simulink model "ESS_3P_2L_220kW_for_LS_Project"  (R2023b)
settings: Solver=VariableStepAuto  StartTime=0.0  StopTime=3  RelTol=1e-3
InitFcn:
  | %Initialization_for_ESS_3P_2L_220kW;
  | Initialization_for_ESS_3P_2L_220kW;
values from neighbouring files (symbols this model uses):
  C_grid = 54e-6    (= 5.4e-05)    [Initialization_for_ESS_3P_2L_220kW.m]    (also in Initialization_for_Testbench.m = 4.5e-05)
  Cdc = 180e-6    (= 0.00018)    [CurrentLoop.m]    (also in Initialization_for_ESS_3P_2L_220kW.m; Initialization_for_Testbench.m)
  Fnom_Grid = 50    [CurrentLoop.m]    (also in Initialization_for_ESS_3P_2L_220kW.m; Initialization_for_Testbench.m)
  Gain_for_ActiveDamping = 1    [Initialization_for_Testbench.m]
  Inom = Pnom/sqrt(3)/Unom_Grid    [CurrentLoop.m]    (also in Initialization_for_ESS_3P_2L_220kW.m; Initialization_for_Testbench.m)
  Ki_Edq = Kp_Edq*2*pi*10    (= 18.8495559215)    [Initialization_for_ESS_3P_2L_220kW.m]
  Ki_Idq = Kp_Idq*2*pi*10    (= 157.913670417)    [Initialization_for_ESS_3P_2L_220kW.m]    (also in Initialization_for_Testbench.m = 1.26330936334)
  Kp_Edq = 0.3    [Initialization_for_ESS_3P_2L_220kW.m]
  Kp_Idq = L_grid*2*pi*2000    (= 2.51327412287)    [Initialization_for_ESS_3P_2L_220kW.m]    (also in Initialization_for_Testbench.m = 2.0106192983)
  L_grid = 200e-6    (= 0.0002)    [Initialization_for_ESS_3P_2L_220kW.m]    (also in Initialization_for_Testbench.m)
  Pnom = 220e3    (= 220000)    [CurrentLoop.m]    (also in Initialization_for_ESS_3P_2L_220kW.m; Initialization_for_Testbench.m = 2500000)
  Ts_Control = 62.5e-6    (= 6.25e-05)    [CurrentLoop.m]    (also in Initialization_for_ESS_3P_2L_220kW.m; Initialization_for_Testbench.m = 0.0001)
  Ts_Power = 10e-7    (= 1e-06)    [Initialization_for_ESS_3P_2L_220kW.m]    (also in Initialization_for_Testbench.m)
  Udc_ref = 1500    [CurrentLoop.m]    (also in Initialization_for_ESS_3P_2L_220kW.m; Initialization_for_Testbench.m)
  Unom_Grid = 690    [CurrentLoop.m]    (also in Initialization_for_ESS_3P_2L_220kW.m; Initialization_for_Testbench.m)
  Unom_Phase = Unom_Grid/sqrt(3)    [CurrentLoop.m]    (also in Initialization_for_ESS_3P_2L_220kW.m; Initialization_for_Testbench.m)
undefined symbols (not defined in the file or in its folder): DiscIntNeverNeededParam, magnitude
libraries: LibraryForCodeGeneration x15, slpidlib x10, spsabctodq0Lib x7, spsAlphaBetaZerotoabcLib x6, simulink x5, spsThreePhaseVIMeasurementLib x4, spsVoltageMeasurementLib x4, eeGeneralControl x3, spsabctoAlphaBetaZeroLib x3, spsSeriesRLCBranchLib x3, spsThreePhaseSeriesRLCBranchLib x3, spsStairGeneratorLib x2
(part 1 of 2)
settings Model: DataDictionary=VariablesDictionary_for_PQ_Control_LCL.sldd  Creator=ZZY  LastModifiedBy=ZZY
settings DataIOCC: ReturnWorkspaceOutputs=off
settings OptimizationCC: UseDivisionForNetSlopeComputation=on

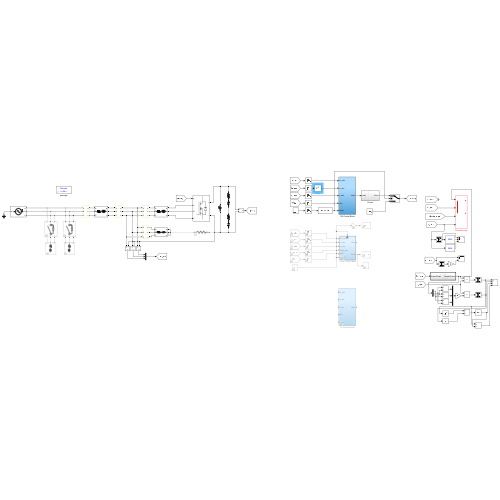
[thumbnail: Simulink's stored preview of the top-level diagram]
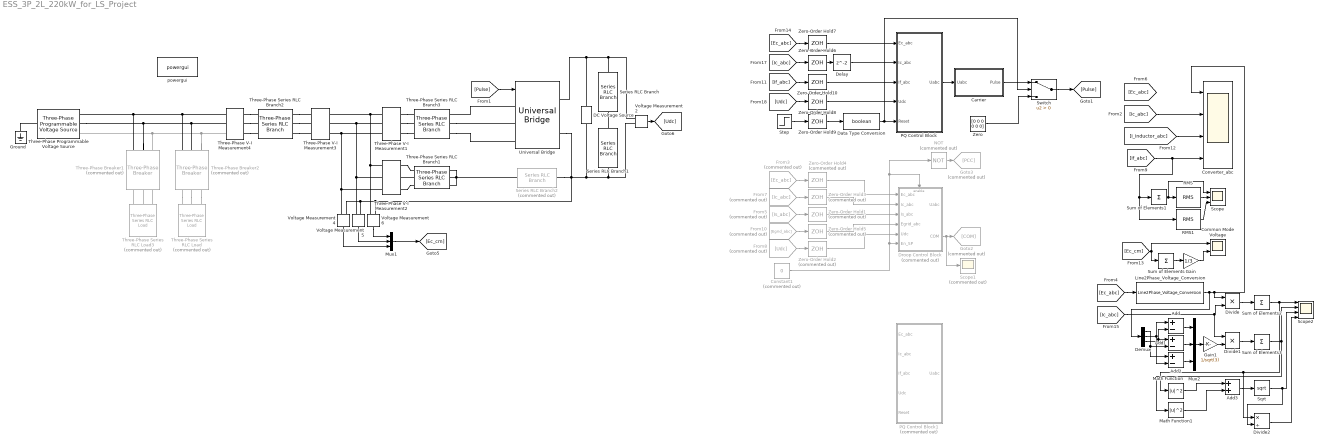
== system ESS_3P_2L_220kW_for_LS_Project ==
  " Droop Control Block" : Subsystem  Commented=on
  " PQ Control Block" : Subsystem
  " PQ Control Block1" : Subsystem  Commented=on
  Add : Sum  Inputs=+-
  Add1 : Sum  Inputs=+-
  Add2 : Sum  Inputs=+-
  Add3 : Sum
  Carrier : Subsystem
  Common Mode Voltage : Scope  NumInputPorts=2
  Constant1 : Constant  Commented=on  Value=0
  Converter_abc : Scope  NumInputPorts=4
  DC Voltage Source : spsDCVoltageSourceLib/DC Voltage Source  Amplitude=Udc_ref  Measurements=None
  Data Type Conversion : DataTypeConversion  OutDataTypeStr=boolean  SaturateOnIntegerOverflow=off  RndMeth=Floor
  Delay : Delay
  Demux : Demux  Outputs=3
  Divide : Product  Inputs=**
  Divide1 : Product  Inputs=**
  Divide2 : Product  Inputs=*/
  From10 : From  Commented=on  GotoTag=Egrid_abc  TagVisibility=global
  From3 : From  Commented=on  GotoTag=Ec_abc  TagVisibility=global
  From5 : From  Commented=on  GotoTag=Is_abc  TagVisibility=global
  From7 : From  Commented=on  GotoTag=Ic_abc  TagVisibility=global
  From8 : From  Commented=on  GotoTag=Udc
  Gain : Gain  Gain=1/3
  Gain1 : Gain  Gain=1/sqrt(3)
  Goto2 : Goto  Commented=on  GotoTag=COM
  Goto3 : Goto  Commented=on  GotoTag=PCC
  Ground : spsGroundLib/Ground  LConnTagsString=a
  Line2Phase_Voltage_Conversion : LibraryForCodeGeneration/Line2Phase_Voltage_Conversion  SystemSampleTime=-1  VariantActivationTime=update diagram  AllowFlexibleInterface=on  Latency=0  AutoFrameSizeCalculation=off
  Math Function : Math  Operator=magnitude^2
  Math Function1 : Math  Operator=magnitude^2
  Mux1 : Mux  Inputs=3
  Mux2 : Mux  Inputs=3
  NOT : Logic  Commented=on  Operator=NOT  IconShape=distinctive  AllPortsSameDT=off  OutDataTypeStr=boolean
  RMS : spsRMSLib/RMS  TrueRMS=on  Freq=100  RMSInit=0  Ts=0
  RMS1 : spsRMSLib/RMS  TrueRMS=on  Freq=10  RMSInit=0  Ts=0
  Scope : Scope  NumInputPorts=3
  Scope1 : Scope  Commented=on
  Scope2 : Scope  NumInputPorts=4
  Series RLC Branch : spsSeriesRLCBranchLib/Series RLC Branch  LConnTagsString=__new0  RConnTagsString=__new0  BranchType=RC  Resistance=1e-3  Inductance=1e-3  SetiL0=off  InitialCurrent=0  Capacitance=Cdc  Setx0=on  InitialVoltage=Udc_ref/3  Measurements=Branch voltage
  Series RLC Branch1 : spsSeriesRLCBranchLib/Series RLC Branch  LConnTagsString=__new0  RConnTagsString=__new0  BranchType=RC  Resistance=100e-3  Inductance=1e-3  SetiL0=off  InitialCurrent=0  Capacitance=Cdc*0.9  Setx0=on  InitialVoltage=Udc_ref/2  Measurements=Branch voltage
  Series RLC Branch2 : spsSeriesRLCBranchLib/Series RLC Branch  Commented=on  LConnTagsString=__new0  RConnTagsString=__new0  BranchType=R  Resistance=1e-6  Inductance=10e-6  SetiL0=off  InitialCurrent=0  Capacitance=Cdc  Setx0=on  InitialVoltage=750  Measurements=Branch voltage
  Sqrt : Sqrt
  Step : Step  Time=0.1  OutDataTypeStr=Inherit: Inherit via back propagation  SampleTime=Ts_Control
  Sum of Elements{,1..3} (4 alike) : Sum  Inputs=+
  Switch : Switch  Criteria=u2 > Threshold  SaturateOnIntegerOverflow=off  InputSameDT=off
  Three-Phase Programmable Voltage Source : spsThreePhaseProgrammableVoltageSourceLib/Three-Phase Programmable Voltage Source  PositiveSequence="[Unom_Grid  0 Fnom_Grid]"  VariationEntity=None  VariationType=Table of time-amplitude pairs  VariationTypeAlt=Step  VariationStep=0.5  VariationRate=10  VariationMagnitude=0.3  VariationFrequency=2  VariationTiming=[1 2]  VariationPhaseA=off  Amplitudes=[1 0.8 1.2 1.0]  TimeValues=[0 0.1 0.15 0.2]  HarmonicGeneration=on  HarmonicA=[1 0.1 45 2]  HarmonicB=[5 0 35 2]  Timing="[1.5  1.7]"  BusType=swing  Pref=0  Qref=0  Qmin=-inf  Qmax=inf
  Three-Phase Series RLC Branch1 : spsThreePhaseSeriesRLCBranchLib/Three-Phase Series RLC Branch  LConnTagsString=A|B|C  RConnTagsString=A|B|C  BranchType=RC  Resistance=1e-3  Inductance=1e-3  Capacitance=C_grid  Measurements=None
  Three-Phase Series RLC Branch2 : spsThreePhaseSeriesRLCBranchLib/Three-Phase Series RLC Branch  LConnTagsString=A|B|C  RConnTagsString=A|B|C  BranchType=RL  Resistance=1e-6  Inductance=L_grid*1e0  Capacitance=1e-6  Measurements=None
  Three-Phase Series RLC Branch3 : spsThreePhaseSeriesRLCBranchLib/Three-Phase Series RLC Branch  LConnTagsString=A|B|C  RConnTagsString=A|B|C  BranchType=RL  Resistance=1e-6  Inductance=L_grid  Capacitance=1e-6  Measurements=None
  Three-Phase Series RLC Load : spsThreePhaseSeriesRLCLoadLib/Three-Phase Series RLC Load  Commented=on  LConnTagsString=A|B|C  Configuration=Delta  NominalVoltage=690  Vabc=[1e3 1e3 1e3]  Vabcp=[1e3 1e3 1e3]  NominalFrequency=50  UnbalancedPower=off  ActivePower=100e3  InductivePower=50e3  CapacitivePower=0  Pabc=[10e3 9e3 11e3]  QLabc=[100 90 110]  QCabc=[100 90 110]  Pabcp=[10e3 9e3 11e3]  QLabcp=[100 90 110]  QCabcp=[100 90 110]  Measurements=None  LoadType=constant Z
  Three-Phase Series RLC Load3 : spsThreePhaseSeriesRLCLoadLib/Three-Phase Series RLC Load  Commented=on  LConnTagsString=A|B|C  Configuration=Delta  NominalVoltage=690  Vabc=[1e3 1e3 1e3]  Vabcp=[1e3 1e3 1e3]  NominalFrequency=50  UnbalancedPower=off  ActivePower=100e3  InductivePower=50e3  CapacitivePower=0  Pabc=[10e3 9e3 11e3]  QLabc=[100 90 110]  QCabc=[100 90 110]  Pabcp=[10e3 9e3 11e3]  QLabcp=[100 90 110]  QCabcp=[100 90 110]  Measurements=None  LoadType=constant Z
  Three-Phase V-I Measurement1 : spsThreePhaseVIMeasurementLib/Three-Phase V-I Measurement  VoltageMeasurement=no  SetLabelV=on  LabelV=Ec_abc  Vpu=off  VpuLL=off  CurrentMeasurement=yes  SetLabelI=on  LabelI=I_inductor_abc  Ipu=off  Pbase=100e6  Vbase=500e3  OutputType=Complex  PhasorSimulation=off  PSBequivalent=0
  Three-Phase V-I Measurement2 : spsThreePhaseVIMeasurementLib/Three-Phase V-I Measurement  VoltageMeasurement=no  SetLabelV=off  LabelV=Ec_abc  Vpu=off  VpuLL=off  CurrentMeasurement=yes  SetLabelI=on  LabelI=If_abc  Ipu=off  Pbase=100e6  Vbase=500e3  OutputType=Complex  PhasorSimulation=off  PSBequivalent=0
  Three-Phase V-I Measurement3 : spsThreePhaseVIMeasurementLib/Three-Phase V-I Measurement  VoltageMeasurement=phase-to-phase  SetLabelV=on  LabelV=Ec_abc  Vpu=off  VpuLL=off  CurrentMeasurement=yes  SetLabelI=on  LabelI=Ic_abc  Ipu=off  Pbase=100e6  Vbase=500e3  OutputType=Complex  PhasorSimulation=off  PSBequivalent=0
  Three-Phase V-I Measurement4 : spsThreePhaseVIMeasurementLib/Three-Phase V-I Measurement  VoltageMeasurement=phase-to-phase  SetLabelV=on  LabelV=Eg_abc  Vpu=off  VpuLL=off  CurrentMeasurement=no  SetLabelI=on  LabelI=Ic_abc  Ipu=off  Pbase=100e6  Vbase=500e3  OutputType=Complex  PhasorSimulation=off  PSBequivalent=0
  Three-Phase Breaker1 : spsThreePhaseBreakerLib/Three-Phase Breaker  Commented=on  InitialState=open  SwitchA=on  SwitchB=on  SwitchC=on  SwitchTimes="[2  6]"  External=off  BreakerResistance=0.01  SnubberResistance=1e6  SnubberCapacitance=inf  Measurements=None
  Three-Phase Breaker2 : spsThreePhaseBreakerLib/Three-Phase Breaker  Commented=on  InitialState=open  SwitchA=on  SwitchB=on  SwitchC=on  SwitchTimes="[4  7]"  External=off  BreakerResistance=0.01  SnubberResistance=1e6  SnubberCapacitance=inf  Measurements=None
  Universal Bridge : spsUniversalBridgeLib/Universal Bridge  Arms=3  SnubberResistance=1e5  SnubberCapacitance=inf  Device=MOSFET / Diodes  Ron=1e-3  Lon=0  ForwardVoltages="[  0  0  ]"  ForwardVoltage=0  GTOparameters=[ 10e-6 , 20e-6 ]  IGBTparameters=[ 1e-6 , 2e-6 ]  Measurements=None  Measurements_2=None  converterType=Rectifier
  Voltage Measurement{2,4..6} (4 alike) : spsVoltageMeasurementLib/Voltage Measurement  PhasorSimulation=off  OutputType=Complex  PSBequivalent=0
  Zero : Constant  Value=[0 0 0 0 0 0]  OutDataTypeStr=Inherit: Inherit via back propagation
  Zero-Order Hold{1..5} (5 alike) : ZeroOrderHold  Commented=on  SampleTime=Ts_Control
  Zero-Order Hold{6..10} (5 alike) : ZeroOrderHold  SampleTime=Ts_Control
  powergui : spspowerguiLib/powergui  Priority=1  SimulationMode=Discrete  SampleTime=Ts_Power  frequency=60  Iterations=50  frequencyindice=50  Pbase=100e6  ErrMax=1e-4  UnitsV=kV  UnitsW=MW  buscounter=0  FunctionMessages=off  echomessages=off  EnableUseOfTLC=off  CurrentSourceSwitches=off  DisableSnubberDevices=off  DisableRonSwitches=off  DisableVfSwitches=off  DisplayEquations=off  AutomaticDiscreteSolvers=off  SolverType=Tustin/Backward Euler (TBE)  Interpol=off  ExternalGateDelay=off  methode=off  Ts=100  x0status=blocks  SPID=on  SwTol=0  HookPort=off  NonlinearTolerance=1e-4  nMaxIteration=100  ContinueOnMaxIteration=off  RestoreLinks=warning  ResistiveCurrentMeasurement=off  Frange=[0:2:500]  Ylog=off  Xlog=on  ShowGrid=off  save=off  variable=ZData  structure=CHB_abc  ZoomFFT=off  StartTime=1.4  cycles=5  DisplayStyle=1  fundamental=50  FreqAxis=off  MaxFrequency=30000  frequencyindicesteady=1  RmsSteady=1  display=off
  wires:
  From3/1 -> Zero-Order Hold4/1
  [Ic_abc] -> Converter_abc/2
  From8/1 -> Zero-Order Hold2/1
  From7/1 -> Zero-Order Hold3/1
  [Pulse] -> Universal Bridge/1
  From5/1 -> Zero-Order Hold1/1
  Zero-Order Hold2/1 -> " Droop Control Block"/5(Udc)
  " Droop Control Block"/2(COM) -> Scope1/1, Goto2/1
  From10/1 -> Zero-Order Hold5/1
  Zero-Order Hold5/1 -> " Droop Control Block"/4(Egrid_abc)
  Zero-Order Hold4/1 -> " Droop Control Block"/1(Ec_abc)
  Zero-Order Hold3/1 -> " Droop Control Block"/2(Ic_abc)
  Zero-Order Hold1/1 -> " Droop Control Block"/3(Is_abc)
  Constant1/1 -> " Droop Control Block"/Enable, NOT/1, " Droop Control Block"/6(En_SP)
  NOT/1 -> Goto3/1
  [Ic_abc] -> Zero-Order Hold6/1
  [Udc] -> Zero-Order Hold8/1
  Zero-Order Hold8/1 -> " PQ Control Block"/4(Udc)
  Step/1 -> Zero-Order Hold9/1
  Switch/1 -> [Pulse]
  Carrier/1(Pulse) -> Switch/1
  Zero/1 -> Switch/3
  Zero-Order Hold9/1 -> Data Type Conversion/1
  Data Type Conversion/1 -> " PQ Control Block"/5(Reset), Switch/2
  [If_abc] -> RMS1/1, Sum of Elements1/1, Converter_abc/4
  [If_abc] -> Zero-Order Hold10/1
  RMS/1 -> Scope/2
  [I_inductor_abc] -> Converter_abc/3
  [Ec_cm] -> Common Mode Voltage/1, Sum of Elements/1
  Sum of Elements/1 -> Gain/1
  Gain/1 -> Common Mode Voltage/2
  Voltage Measurement4/1 -> Mux1/3
  Mux1/1 -> [Ec_cm]
  Voltage Measurement6/1 -> Mux1/1
  Voltage Measurement5/1 -> Mux1/2
  " PQ Control Block"/1(Uabc) -> Carrier/1(Uabc)
  Sum of Elements1/1 -> Scope/1, RMS/1
  Voltage Measurement2/1 -> [Udc]
  Zero-Order Hold7/1 -> " PQ Control Block"/1(Ec_abc)
  RMS1/1 -> Scope/3
  [Ec_abc] -> Zero-Order Hold7/1
  [Ec_abc] -> Line2Phase_Voltage_Conversion/1
  [Ic_abc] -> Divide1/1, Divide/2
  Divide/1 -> Sum of Elements2/1
  Sum of Elements2/1 -> Divide2/1, Math Function/1, Scope2/1
  Line2Phase_Voltage_Conversion/1 -> Converter_abc/1, Divide/1, Demux/1
  Gain1/1 -> Divide1/2
  Divide1/1 -> Sum of Elements3/1
  Sum of Elements3/1 -> Scope2/2, Math Function1/1
  Mux2/1 -> Gain1/1
  Add/1 -> Mux2/1
  Add1/1 -> Mux2/2
  Add2/1 -> Mux2/3
  Demux/2 -> Add2/2, Add/1
  Demux/3 -> Add1/1, Add/2
  Demux/1 -> Add2/1, Add1/2
  Math Function/1 -> Add3/1
  Math Function1/1 -> Add3/2
  Add3/1 -> Sqrt/1
  Divide2/1 -> Scope2/4
  Sqrt/1 -> Divide2/2, Scope2/3
  Zero-Order Hold10/1 -> " PQ Control Block"/3(If_abc)
  Zero-Order Hold6/1 -> Delay/1
  Delay/1 -> " PQ Control Block"/2(Ic_abc)
  connections:
  Three-Phase V-I Measurement1/LConn1 -- Three-Phase V-I Measurement2/LConn1 -- Voltage Measurement6/LConn1 -- Three-Phase V-I Measurement3/RConn1
  Three-Phase V-I Measurement1/LConn2 -- Three-Phase V-I Measurement2/LConn2 -- Voltage Measurement5/LConn1 -- Three-Phase V-I Measurement3/RConn2
  Three-Phase V-I Measurement1/LConn3 -- Three-Phase V-I Measurement2/LConn3 -- Voltage Measurement4/LConn1 -- Three-Phase V-I Measurement3/RConn3
  Series RLC Branch/LConn1 -- DC Voltage Source/RConn1 -- Universal Bridge/RConn1 -- Voltage Measurement2/LConn1
  Three-Phase Series RLC Load3/LConn1 -- Three-Phase Breaker1/LConn1
  Three-Phase Series RLC Load3/LConn2 -- Three-Phase Breaker1/LConn2
  Three-Phase Series RLC Load3/LConn3 -- Three-Phase Breaker1/LConn3
  Three-Phase V-I Measurement1/RConn1 -- Three-Phase Series RLC Branch3/LConn1
  Three-Phase V-I Measurement1/RConn2 -- Three-Phase Series RLC Branch3/LConn2
  Three-Phase V-I Measurement1/RConn3 -- Three-Phase Series RLC Branch3/LConn3
  Three-Phase Breaker2/RConn3 -- Three-Phase Breaker1/RConn3 -- Three-Phase Programmable Voltage Source/RConn3 -- Three-Phase V-I Measurement4/LConn3
  Three-Phase V-I Measurement4/LConn2 -- Three-Phase Breaker2/RConn2 -- Three-Phase Programmable Voltage Source/RConn2 -- Three-Phase Breaker1/RConn2
  Three-Phase Breaker2/RConn1 -- Three-Phase V-I Measurement4/LConn1 -- Three-Phase Breaker1/RConn1 -- Three-Phase Programmable Voltage Source/RConn1
  Three-Phase Breaker2/LConn1 -- Three-Phase Series RLC Load/LConn1
  Three-Phase Breaker2/LConn2 -- Three-Phase Series RLC Load/LConn2
  Three-Phase Breaker2/LConn3 -- Three-Phase Series RLC Load/LConn3
  Three-Phase Series RLC Branch1/LConn2 -- Three-Phase V-I Measurement2/RConn2
  Three-Phase V-I Measurement2/RConn1 -- Three-Phase Series RLC Branch1/LConn1
  Three-Phase V-I Measurement2/RConn3 -- Three-Phase Series RLC Branch1/LConn3
  Three-Phase Series RLC Branch1/RConn1 -- Series RLC Branch2/LConn1 -- Three-Phase Series RLC Branch1/RConn2 -- Three-Phase Series RLC Branch1/RConn3
  Three-Phase Series RLC Branch2/RConn1 -- Three-Phase V-I Measurement3/LConn1
  Three-Phase Series RLC Branch2/RConn2 -- Three-Phase V-I Measurement3/LConn2
  Three-Phase Series RLC Branch2/RConn3 -- Three-Phase V-I Measurement3/LConn3
  Three-Phase V-I Measurement4/RConn1 -- Three-Phase Series RLC Branch2/LConn1
  Three-Phase V-I Measurement4/RConn2 -- Three-Phase Series RLC Branch2/LConn2
  Three-Phase V-I Measurement4/RConn3 -- Three-Phase Series RLC Branch2/LConn3
  Three-Phase Series RLC Branch3/RConn2 -- Universal Bridge/LConn2
  Universal Bridge/LConn1 -- Three-Phase Series RLC Branch3/RConn1
  Three-Phase Series RLC Branch3/RConn3 -- Universal Bridge/LConn3
  Voltage Measurement4/LConn2 -- Voltage Measurement5/LConn2 -- Voltage Measurement6/LConn2 -- Series RLC Branch1/RConn1 -- Voltage Measurement2/LConn2 -- DC Voltage Source/LConn1 -- Series RLC Branch2/RConn1 -- Universal Bridge/RConn2
  Series RLC Branch1/LConn1 -- Series RLC Branch/RConn1
  Ground/LConn1 -- Three-Phase Programmable Voltage Source/LConn1

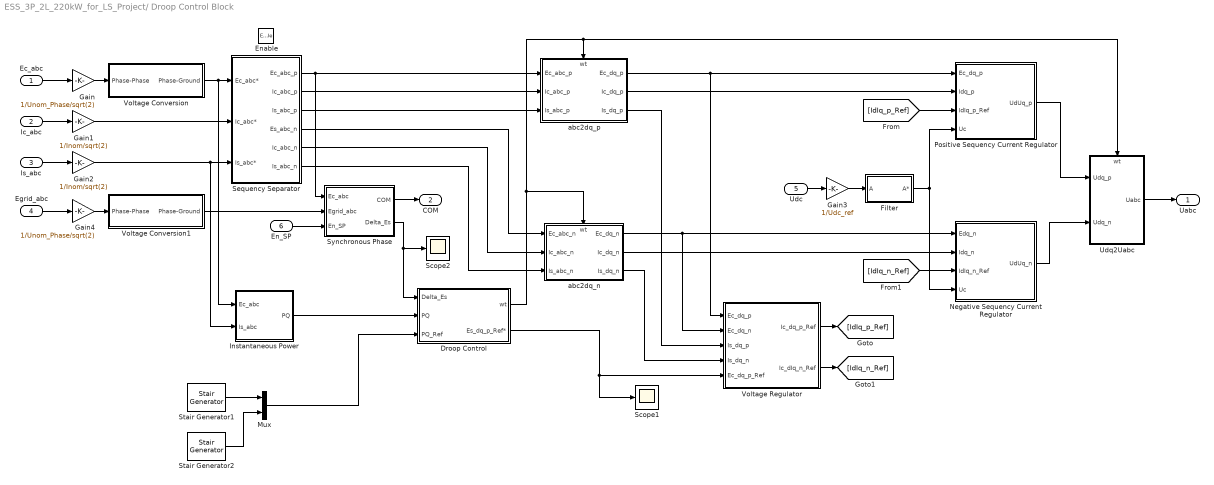
== system ESS_3P_2L_220kW_for_LS_Project/ Droop Control Block ==
  Ec_abc : Inport
  Ic_abc : Inport  Port=2
  Is_abc : Inport  Port=3
  Egrid_abc : Inport  Port=4
  Udc : Inport  Port=5
  En_SP : Inport  Port=6
  Enable : EnablePort
  Droop Control : Subsystem
  Filter : Subsystem
  Gain : Gain  Gain=1/Unom_Phase/sqrt(2)
  Gain1 : Gain  Gain=1/Inom/sqrt(2)
  Gain2 : Gain  Gain=1/Inom/sqrt(2)
  Gain3 : Gain  Gain=1/Udc_ref
  Gain4 : Gain  Gain=1/Unom_Phase/sqrt(2)
  Instantaneous Power : Subsystem
  Mux : Mux  Inputs=2
  Negative Sequency Current Regulator : Subsystem
  Positive Sequency Current Regulator : Subsystem
  Scope1 : Scope
  Scope2 : Scope
  Sequency Separator : Subsystem
  Stair Generator1 : spsStairGeneratorLib/Stair Generator  t=[0, 2, 4, 6, 8]  e=[0, -0.909/2,-0.909, -0.909/2, 0]  Ts=0
  Stair Generator2 : spsStairGeneratorLib/Stair Generator  t=[0, 2, 4, 6, 8]  e=[0, -0.45/2, -0.45, -0.45/2, 0]  Ts=0
  Synchronous Phase : Subsystem
  Udq2Uabc : Subsystem
      settings: PortSchema="{\"entries\":[{\"content\":{\"sides\":[{\"content\":{\"connectorIds\":[\"In1\",\"In2\"]},\"type\":\"ConnectorPlacement.EquallySpacedRectSide\",\"uuid\":\"009786f4-728c-4160-b9bf-eaf0b5a05101\"},{\"content\":{\"connectorIds\":[\"Out1\"],\"side\":\"RIGHT\"},\"type\":\"ConnectorPlacement.EquallySpacedRectSide\",\"uuid\":\"2a94367a-5c57-4632-9573-ab089470159a\"},{\"content\":{\"connectorIds\":[\"In3\"],\"side\":\"TOP\"},\"type\":\"ConnectorPlacement.EquallySpacedRectSide\",\"uuid\":\"6906365b-3187-4c4b-97cf-c9dec4c5ef7c\"}]},\"type\":\"ConnectorPlacement.EquallySpacedConnector\",\"uuid\":\"96ca8566-a266-405c-817a-b47b433d51ed\"}],\"packageUris\":[\"http://schema.mathworks.com/mf0/Connector/R2020b\"],\"version\":\"1.0\"}"
  Voltage Conversion : Subsystem
  Voltage Conversion1 : Subsystem
  Voltage Regulator : Subsystem
  abc2dq_n : Subsystem
      settings: PortSchema="{\"entries\":[{\"content\":{\"sides\":[{\"content\":{\"connectorIds\":[\"In1\",\"In2\",\"In3\"]},\"type\":\"ConnectorPlacement.EquallySpacedRectSide\",\"uuid\":\"609992f3-b9d4-4332-9f12-3698389607f5\"},{\"content\":{\"connectorIds\":[\"Out1\",\"Out2\",\"Out3\"],\"side\":\"RIGHT\"},\"type\":\"ConnectorPlacement.EquallySpacedRectSide\",\"uuid\":\"e927e70d-df4f-4429-acad-b4b457f9cd78\"},{\"content\":{\"connectorIds\":[\"In4\"],\"side\":\"TOP\"},\"type\":\"ConnectorPlacement.EquallySpacedRectSide\",\"uuid\":\"705909b5-5303-4c1a-bc4d-057cb742f6aa\"}]},\"type\":\"ConnectorPlacement.EquallySpacedConnector\",\"uuid\":\"c16fd8e1-129c-40cf-a015-8bc920263e1d\"}],\"packageUris\":[\"http://schema.mathworks.com/mf0/Connector/R2020b\"],\"version\":\"1.0\"}"
  abc2dq_p : Subsystem
      settings: PortSchema="{\"entries\":[{\"content\":{\"sides\":[{\"content\":{\"connectorIds\":[\"In1\",\"In2\",\"In3\"]},\"type\":\"ConnectorPlacement.EquallySpacedRectSide\",\"uuid\":\"da265cd8-5bbd-481b-835e-96e26ace7bfd\"},{\"content\":{\"connectorIds\":[\"Out1\",\"Out2\",\"Out3\"],\"side\":\"RIGHT\"},\"type\":\"ConnectorPlacement.EquallySpacedRectSide\",\"uuid\":\"df43d14a-96c1-4a1d-9f34-3d0fd032842c\"},{\"content\":{\"connectorIds\":[\"In4\"],\"side\":\"TOP\"},\"type\":\"ConnectorPlacement.EquallySpacedRectSide\",\"uuid\":\"67136f89-5f84-4cef-96c4-01ffaabf096c\"}]},\"type\":\"ConnectorPlacement.EquallySpacedConnector\",\"uuid\":\"98978efc-5647-482c-8e21-5c69e1d08dbc\"}],\"packageUris\":[\"http://schema.mathworks.com/mf0/Connector/R2020b\"],\"version\":\"1.0\"}"
  Uabc : Outport
  COM : Outport  Port=2
  wires:
  Sequency Separator/6(Is_abc_n) -> abc2dq_n/3(Is_abc_n)
  Sequency Separator/3(Is_abc_p) -> abc2dq_p/3(Is_abc_p)
  Gain2/1 -> Instantaneous Power/2(Is_abc), Sequency Separator/3(Is_abc*)
  Is_abc/1 -> Gain2/1
  Negative Sequency Current Regulator/1(UdUq_n) -> Udq2Uabc/2(Udq_n)
  Positive Sequency Current Regulator/1(UdUq_p) -> Udq2Uabc/1(Udq_p)
  Filter/1(A*) -> Positive Sequency Current Regulator/4(Uc), Negative Sequency Current Regulator/4(Uc)
  Udq2Uabc/1(Uabc) -> Uabc/1
  Sequency Separator/2(Ic_abc_p) -> abc2dq_p/2("Ic_abc_p ")
  abc2dq_p/2(Ic_dq_p) -> Positive Sequency Current Regulator/2(Idq_p)
  Gain1/1 -> Sequency Separator/2(" Ic_abc*")
  Gain3/1 -> Filter/1(A)
  abc2dq_n/2(Ic_dq_n) -> Negative Sequency Current Regulator/2(Idq_n)
  Sequency Separator/1(Ec_abc_p) -> abc2dq_p/1(Ec_abc_p), Synchronous Phase/1(Ec_abc)
  Udc/1 -> Gain3/1
  Sequency Separator/5(Ic_abc_n) -> abc2dq_n/2("Ic_abc_n ")
  Sequency Separator/4(Es_abc_n) -> abc2dq_n/1(Ec_abc_n)
  abc2dq_n/1(Ec_dq_n) -> Voltage Regulator/2(Ec_dq_n), Negative Sequency Current Regulator/1(Edq_n)
  [IdIq_n_Ref] -> Negative Sequency Current Regulator/3(IdIq_n_Ref)
  Voltage Conversion/1(Phase-Ground) -> Instantaneous Power/1(Ec_abc), Sequency Separator/1(Ec_abc*)
  Gain/1 -> Voltage Conversion/1(Phase-Phase)
  abc2dq_p/1(Ec_dq_p) -> Positive Sequency Current Regulator/1(Ec_dq_p), Voltage Regulator/1(Ec_dq_p)
  [IdIq_p_Ref] -> Positive Sequency Current Regulator/3(IdIq_p_Ref)
  Ic_abc/1 -> Gain1/1
  Ec_abc/1 -> Gain/1
  Voltage Regulator/1(Ic_dq_p_Ref) -> [IdIq_p_Ref]
  Voltage Regulator/2(Ic_dIq_n_Ref) -> [IdIq_n_Ref]
  abc2dq_p/3(Is_dq_p) -> Voltage Regulator/3(Is_dq_p)
  Droop Control/2(Es_dq_p_Ref*) -> Scope1/1, Voltage Regulator/5(Ec_dq_p_Ref)
  Droop Control/1(wt) -> Udq2Uabc/3(wt), abc2dq_p/4(wt), abc2dq_n/4(wt)
  Instantaneous Power/1(PQ) -> Droop Control/2(PQ)
  Egrid_abc/1 -> Gain4/1
  Gain4/1 -> Voltage Conversion1/1(Phase-Phase)
  Synchronous Phase/1(COM) -> COM/1
  abc2dq_n/3(Is_dq_n) -> Voltage Regulator/4(Is_dq_n)
  Voltage Conversion1/1(Phase-Ground) -> Synchronous Phase/2(Egrid_abc)
  Mux/1 -> Droop Control/3(PQ_Ref)
  Synchronous Phase/2(Delta_Es) -> Droop Control/1(Delta_Es), Scope2/1
  Stair Generator1/1 -> Mux/1
  Stair Generator2/1 -> Mux/2
  En_SP/1 -> Synchronous Phase/3(En_SP)

== system ESS_3P_2L_220kW_for_LS_Project/ PQ Control Block ==
  Ec_abc : Inport
  Ic_abc : Inport  Port=2
  If_abc : Inport  Port=3
  Udc : Inport  Port=4
  Reset : Inport  Port=5  OutDataTypeStr=boolean
  Data Type Conversion{,1..4} (5 alike) : DataTypeConversion  OutDataTypeStr=single  RndMeth=Nearest  SaturateOnIntegerOverflow=off
  Data Type Conversion5 : DataTypeConversion  OutDataTypeStr=double  RndMeth=Nearest  SaturateOnIntegerOverflow=off
  Gain1 : Gain  Gain=220000
  Model : ModelReference  ModelNameDialog=PQ_Control_LCL.slx  SimulationMode=Normal  ModelReferenceVersion=1.120
  Mux : Mux  Inputs=2
  Stair Generator1 : eeStairGenerator/Stair Generator  LabelModeActiveChoice=Discrete  TimeInput=0:0.5:2.5  AmplitudeInput=0:0.2:1  SampleTime=Ts_Control  RepeatPattern=off  OutDataTypeStr=double
      settings: LibrarySourceBlock=ee_sl_lib/General Control/Stair Generator
  Zero : Constant  Value=0  OutDataTypeStr=Inherit: Inherit via back propagation
  Uabc : Outport
  wires:
  Ec_abc/1 -> Data Type Conversion/1
  Ic_abc/1 -> Data Type Conversion1/1
  Udc/1 -> Data Type Conversion2/1
  Model/1 -> Data Type Conversion5/1
  Stair Generator1/1 -> Mux/1
  Zero/1 -> Mux/2
  Data Type Conversion/1 -> Model/1
  Data Type Conversion1/1 -> Model/2
  Data Type Conversion5/1 -> Uabc/1
  Reset/1 -> Model/6
  Mux/1 -> Gain1/1
  Data Type Conversion3/1 -> Model/5
  Data Type Conversion2/1 -> Model/4
  Gain1/1 -> Data Type Conversion3/1
  If_abc/1 -> Data Type Conversion4/1
  Data Type Conversion4/1 -> Model/3

== system ESS_3P_2L_220kW_for_LS_Project/ PQ Control Block1 ==
  Ec_abc : Inport
  Ic_abc : Inport  Port=2
  If_abc : Inport  Port=3
  Udc : Inport  Port=4
  Reset : Inport  Port=5  OutDataTypeStr=boolean
  Data Type Conversion{,1..4} (5 alike) : DataTypeConversion  OutDataTypeStr=single  RndMeth=Nearest  SaturateOnIntegerOverflow=off
  Data Type Conversion5 : DataTypeConversion  OutDataTypeStr=double  RndMeth=Nearest  SaturateOnIntegerOverflow=off
  Gain1 : Gain  Gain=220000
  Mux : Mux  Inputs=2
  Stair Generator1 : eeStairGenerator/Stair Generator  LabelModeActiveChoice=Discrete  TimeInput=0:0.25:1.25  AmplitudeInput=0:0.2:1  SampleTime=Ts_Control  RepeatPattern=off  OutDataTypeStr=double
      settings: LibrarySourceBlock=ee_sl_lib/General Control/Stair Generator
  Subsystem : Subsystem  TreatAsAtomicUnit=on  SystemSampleTime=Ts_Control
  Zero : Constant  Value=0  OutDataTypeStr=Inherit: Inherit via back propagation
  Uabc : Outport
  wires:
  Ec_abc/1 -> Data Type Conversion/1
  Ic_abc/1 -> Data Type Conversion1/1
  Udc/1 -> Data Type Conversion2/1
  Subsystem/1(Mabc) -> Data Type Conversion5/1
  Stair Generator1/1 -> Mux/1
  Zero/1 -> Mux/2
  Data Type Conversion/1 -> Subsystem/1(Ec_abc)
  Data Type Conversion1/1 -> Subsystem/2(Ic_abc)
  Data Type Conversion5/1 -> Uabc/1
  Reset/1 -> Subsystem/6(Reset)
  Mux/1 -> Gain1/1
  Data Type Conversion3/1 -> Subsystem/5(PQ_Ref)
  Data Type Conversion2/1 -> Subsystem/4(Udc)
  Gain1/1 -> Data Type Conversion3/1
  If_abc/1 -> Data Type Conversion4/1
  Data Type Conversion4/1 -> Subsystem/3(If_abc)

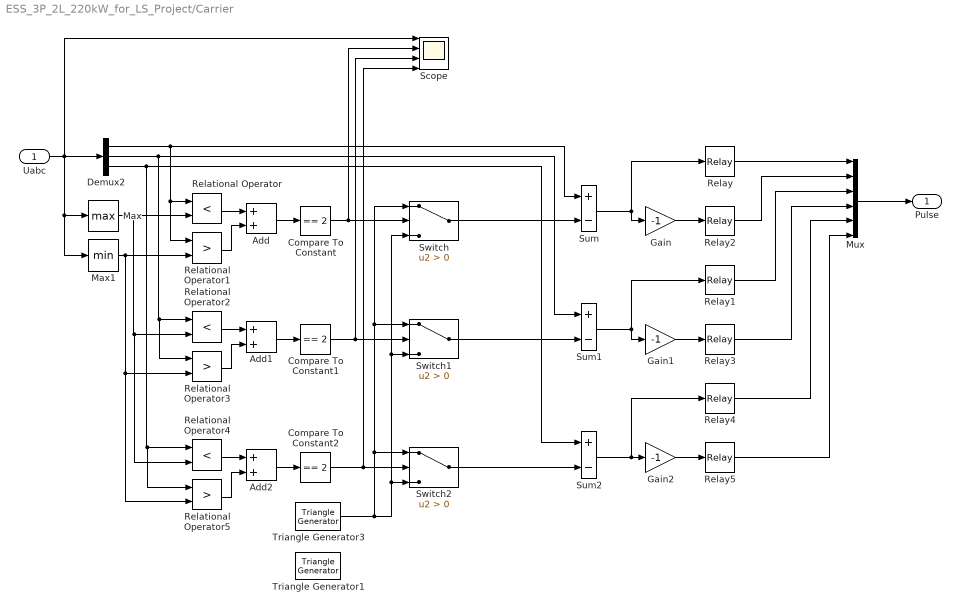
== system ESS_3P_2L_220kW_for_LS_Project/Carrier ==
  Uabc : Inport
  Add : Sum
  Add1 : Sum
  Add2 : Sum
  Compare To Constant : simulink/Logic and Bit Operations/Compare To Constant  relop===  const=2  OutDataTypeStr=boolean
  Compare To Constant1 : simulink/Logic and Bit Operations/Compare To Constant  relop===  const=2  OutDataTypeStr=boolean
  Compare To Constant2 : simulink/Logic and Bit Operations/Compare To Constant  relop===  const=2  OutDataTypeStr=boolean
  Demux2 : Demux  Outputs=3
  Gain : Gain  Gain=-1
  Gain1 : Gain  Gain=-1
  Gain2 : Gain  Gain=-1
  Max : MinMax  Function=max
  Max1 : MinMax
  Mux : Mux  Inputs=6
  Relational Operator : RelationalOperator  Operator=<  OutDataTypeStr=boolean  RndMeth=Simplest  InputSameDT=off
  Relational Operator1 : RelationalOperator  Operator=>  OutDataTypeStr=boolean  RndMeth=Simplest  InputSameDT=off
  Relational Operator2 : RelationalOperator  Operator=<  OutDataTypeStr=boolean  RndMeth=Simplest  InputSameDT=off
  Relational Operator3 : RelationalOperator  Operator=>  OutDataTypeStr=boolean  RndMeth=Simplest  InputSameDT=off
  Relational Operator4 : RelationalOperator  Operator=<  OutDataTypeStr=boolean  RndMeth=Simplest  InputSameDT=off
  Relational Operator5 : RelationalOperator  Operator=>  OutDataTypeStr=boolean  RndMeth=Simplest  InputSameDT=off
  Relay{,1..5} (6 alike) : Relay  OffSwitchValue=-eps
  Scope : Scope  NumInputPorts=4
  Sum : Sum  Inputs=+-
  Sum1 : Sum  Inputs=+-
  Sum2 : Sum  Inputs=+-
  Switch : Switch  Criteria=u2 > Threshold  SaturateOnIntegerOverflow=off  InputSameDT=off
  Switch1 : Switch  Criteria=u2 > Threshold  SaturateOnIntegerOverflow=off  InputSameDT=off
  Switch2 : Switch  Criteria=u2 > Threshold  SaturateOnIntegerOverflow=off  InputSameDT=off
  Triangle Generator1 : spsTriangleGeneratorLib/Triangle Generator  Freq=16000  Phase=0  Ts=1e-6
  Triangle Generator3 : spsTriangleGeneratorLib/Triangle Generator  Freq=16000  Phase=180  Ts=1e-6
  Pulse : Outport
  wires:
  Mux/1 -> Pulse/1
  Gain/1 -> Relay2/1
  Sum/1 -> Relay/1, Gain/1
  Switch/1 -> Sum/2
  Uabc/1 -> Scope/1, Max1/1, Max/1, Demux2/1
  Demux2/1 -> Sum/1, Relational Operator1/1, Relational Operator/1
  Relay/1 -> Mux/1
  Relay2/1 -> Mux/2
  Relay1/1 -> Mux/3
  Relay3/1 -> Mux/4
  Gain1/1 -> Relay3/1
  Demux2/2 -> Relational Operator3/1, Relational Operator2/1, Sum1/1
  Sum1/1 -> Relay1/1, Gain1/1
  Switch1/1 -> Sum1/2
  Relay5/1 -> Mux/6
  Demux2/3 -> Relational Operator5/1, Relational Operator4/1, Sum2/1
  Gain2/1 -> Relay5/1
  Sum2/1 -> Relay4/1, Gain2/1
  Switch2/1 -> Sum2/2
  Relay4/1 -> Mux/5
  Triangle Generator3/1 -> Switch2/3, Switch1/3, Switch/3, Switch/1, Switch1/1, Switch2/1
  Compare To Constant/1 -> Scope/2, Switch/2
  Compare To Constant1/1 -> Scope/3, Switch1/2
  Compare To Constant2/1 -> Scope/4, Switch2/2
  Add/1 -> Compare To Constant/1
  Add1/1 -> Compare To Constant1/1
  Add2/1 -> Compare To Constant2/1
  Relational Operator/1 -> Add/1
  Relational Operator1/1 -> Add/2
  Max/1 -> Relational Operator4/2, Relational Operator2/2, Relational Operator/2
  Max1/1 -> Relational Operator5/2, Relational Operator3/2, Relational Operator1/2
  Relational Operator2/1 -> Add1/1
  Relational Operator3/1 -> Add1/2
  Relational Operator4/1 -> Add2/1
  Relational Operator5/1 -> Add2/2

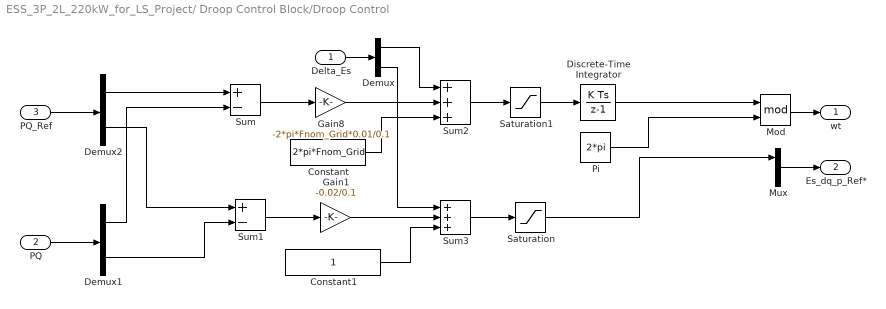
== system ESS_3P_2L_220kW_for_LS_Project/ Droop Control Block/Droop Control ==
  Delta_Es : Inport
  PQ : Inport  Port=2
  PQ_Ref : Inport  Port=3
  Constant : Constant  Value=2*pi*Fnom_Grid
  Constant1 : Constant
  Demux : Demux  Outputs=2
  Demux1 : Demux  Outputs=2
  Demux2 : Demux  Outputs=2
  Discrete-Time Integrator : DiscreteIntegrator  gainval=1  SampleTime=Ts_Control  ICPrevOutput=DiscIntNeverNeededParam  ICPrevScaledInput=DiscIntNeverNeededParam
  Gain1 : Gain  Gain=-0.02/0.1
  Gain8 : Gain  Gain=-2*pi*Fnom_Grid*0.01/0.1
  Mod : Math  Operator=mod
  Mux : Mux  Inputs=2
  Pi : Constant  Value=2*pi  OutDataTypeStr=Inherit: Inherit via back propagation
  Saturation : Saturate  UpperLimit=2  LowerLimit=0.8
  Saturation1 : Saturate  UpperLimit=2*pi*Fnom_Grid*2  LowerLimit=2*pi*Fnom_Grid*0.9
  Sum : Sum  Inputs=+-  InputSameDT=on  SaturateOnIntegerOverflow=on  OutDataTypeStr=Inherit: Same as first input
  Sum1 : Sum  Inputs=+-  InputSameDT=on  SaturateOnIntegerOverflow=on  OutDataTypeStr=Inherit: Same as first input
  Sum2 : Sum  Inputs=+++  InputSameDT=on  SaturateOnIntegerOverflow=on  OutDataTypeStr=Inherit: Same as first input
  Sum3 : Sum  Inputs=+++  InputSameDT=on  SaturateOnIntegerOverflow=on  OutDataTypeStr=Inherit: Same as first input
  wt : Outport
  Es_dq_p_Ref* : Outport  Port=2
  wires:
  PQ_Ref/1 -> Demux2/1
  PQ/1 -> Demux1/1
  Demux2/1 -> Sum/1
  Demux1/1 -> Sum/2
  Demux2/2 -> Sum1/1
  Demux1/2 -> Sum1/2
  Sum/1 -> Gain8/1
  Sum1/1 -> Gain1/1
  Constant/1 -> Sum2/3
  Gain1/1 -> Sum3/2
  Constant1/1 -> Sum3/3
  Sum3/1 -> Saturation/1
  Sum2/1 -> Saturation1/1
  Gain8/1 -> Sum2/2
  Mod/1 -> wt/1
  Pi/1 -> Mod/2
  Delta_Es/1 -> Demux/1
  Demux/2 -> Sum3/1
  Mux/1 -> Es_dq_p_Ref*/1
  Saturation/1 -> Mux/1
  Saturation1/1 -> Discrete-Time Integrator/1
  Discrete-Time Integrator/1 -> Mod/1
  Demux/1 -> Sum2/1

== system ESS_3P_2L_220kW_for_LS_Project/ Droop Control Block/Filter ==
  A : Inport
  A* : Outport
  wires:
  A/1 -> A*/1

== system ESS_3P_2L_220kW_for_LS_Project/ Droop Control Block/Instantaneous Power ==
  Ec_abc : Inport
  Is_abc : Inport  Port=2
  Add : Sum  Inputs=+-
  Add1 : Sum  Inputs=+-
  Add2 : Sum  Inputs=+-
  Demux : Demux  Outputs=3
  Dot Product : DotProduct  OutDataTypeStr=Inherit: Inherit via internal rule
  Dot Product1 : DotProduct  OutDataTypeStr=Inherit: Inherit via internal rule
  Gain : Gain  Gain=1/sqrt(3)
  Gain4 : Gain  Gain=2/3
  Moving Average : eeGeneralControl/Moving Average  VariantControl=Variant1  LabelModeActiveChoice=Discrete  f=Fnom_Grid*1  x0=0  BufferSize=8192  Ts=Ts_Control
      settings: LibrarySourceBlock=ee_sl_lib/General Control/Moving Average
  Mux : Mux  Inputs=2
  Mux1 : Mux  Inputs=3
  Scope1 : Scope  NumInputPorts=2
  PQ : Outport
  wires:
  Ec_abc/1 -> Demux/1, Dot Product/1
  Is_abc/1 -> Dot Product/2, Dot Product1/2
  Mux/1 -> Gain4/1
  Dot Product/1 -> Mux/1
  Demux/2 -> Add2/2, Add/1
  Demux/3 -> Add1/1, Add/2
  Demux/1 -> Add2/1, Add1/2
  Add/1 -> Mux1/1
  Add1/1 -> Mux1/2
  Add2/1 -> Mux1/3
  Mux1/1 -> Dot Product1/1
  Dot Product1/1 -> Gain/1
  Gain/1 -> Mux/2
  Gain4/1 -> Scope1/1, Moving Average/1
  Moving Average/1 -> Scope1/2, PQ/1

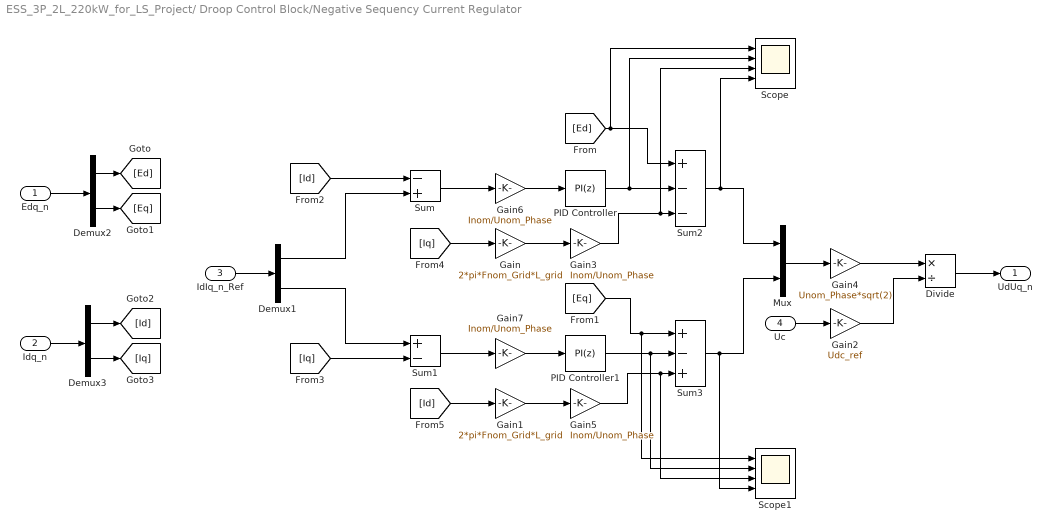
== system ESS_3P_2L_220kW_for_LS_Project/ Droop Control Block/Negative Sequency Current Regulator ==
  Edq_n : Inport
  Idq_n : Inport  Port=2
  IdIq_n_Ref : Inport  Port=3  PortDimensions=2
  Uc : Inport  Port=4
  Demux1 : Demux  Outputs=2
  Demux2 : Demux  Outputs=2
  Demux3 : Demux  Outputs=2
  Divide : Product  Inputs=*/
  Gain : Gain  Gain=2*pi*Fnom_Grid*L_grid
  Gain1 : Gain  Gain=2*pi*Fnom_Grid*L_grid
  Gain2 : Gain  Gain=Udc_ref
  Gain{3,5..7} (4 alike) : Gain  Gain=Inom/Unom_Phase
  Gain4 : Gain  Gain=Unom_Phase*sqrt(2)
  Mux : Mux  Inputs=2
  PID Controller : slpidlib/PID Controller  Controller=PI  Form=Parallel  TimeDomain=Discrete-time  UseExternalTs=off  SampleTime=Ts_Control  IntegratorMethod=Forward Euler  FilterMethod=Forward Euler  ControllerParametersSource=internal  P=Kp_Idq  I=Ki_Idq  UseKiTs=off  D=0  N=100  UseFilter=on  TunerSelectOption=Transfer Function Based (PID Tuner App)  InitialConditionSource=internal  InitialConditionForIntegrator=0  InitialConditionForFilter=0  DifferentiatorICPrevScaledInput=0  ExternalReset=none  TrackingMode=off  Kt=1  LimitOutput=on  SatLimitsSource=internal  UpperSaturationLimit=4  LowerSaturationLimit=-4  LinearizeAsGain=on  AntiWindupMode=clamping  Kb=1  LimitIntegrator=off  UpperIntegratorSaturationLimit=inf  LowerIntegratorSaturationLimit=-inf  POutMin=[]  POutMax=[]  IOutMin=[]  IOutMax=[]  DOutMin=[]  DOutMax=[]  NOutMin=[]  NOutMax=[]  SumOutMin=[]  SumOutMax=[]  SaturationOutMin=[]  SaturationOutMax=[]  PParamMin=[]  PParamMax=[]  IParamMin=[]  IParamMax=[]  DParamMin=[]  DParamMax=[]  NParamMin=[]  NParamMax=[]  KbParamMin=[]  KbParamMax=[]  KtParamMin=[]  KtParamMax=[]  KbOutMin=[]  KbOutMax=[]  KtOutMin=[]  KtOutMax=[]  IntegratorOutMin=[]  IntegratorOutMax=[]  FilterOutMin=[]  FilterOutMax=[]  SumI1OutMin=[]  SumI1OutMax=[]  SumI2OutMin=[]  SumI2OutMax=[]  SumI3OutMin=[]  SumI3OutMax=[]  SumI4OutMin=[]  SumI4OutMax=[]  SumDOutMin=[]  SumDOutMax=[]  DifferentiatorOutMin=[]  DifferentiatorOutMax=[]  FilterDiffOutCoefMin=[]  FilterDiffOutCoefMax=[]  ReciprocalOutMin=[]  ReciprocalOutMax=[]  SumDenOutMin=[]  SumDenOutMax=[]  SumNumOutMin=[]  SumNumOutMax=[]  DivideOutMin=[]  DivideOutMax=[]  UdiffTsProdOutMin=[]  UdiffTsProdOutMax=[]  NTsProdOutMin=[]  NTsProdOutMax=[]  UintegralTsProdOutMin=[]  UintegralTsProdOutMax=[]  UngainTsProdOutMin=[]  UngainTsProdOutMax=[]  ClampingZeroOutDataTypeStr=Inherit: Inherit via back propagation  ClampingZeroOutMin=[]  ClampingZeroOutMax=[]  FilterDenConstantOutDataTypeStr=Inherit: Inherit via back propagation  FilterDenConstantOutMin=[]  FilterDenConstantOutMax=[]  PCopyOutDataTypeStr=Inherit: Inherit via back propagation  PCopyOutMin=[]  PCopyOutMax=[]  NCopyOutDataTypeStr=Inherit: Inherit via back propagation  NCopyOutMin=[]  NCopyOutMax=[]  IntegratorContinuousStateAttributes=''  IntegratorStateMustResolveToSignalObject=off  IntegratorRTWStateStorageClass=Auto  FilterContinuousStateAttributes=''  FilterStateMustResolveToSignalObject=off  FilterRTWStateStorageClass=Auto  ParallelPVariant=InternalParameters  IdealPVariant=Disabled  IVariant=InternalParameters  DVariant=Disabled  IntegratorVariant=Discrete  SatVariant=Enabled  AWVariant=DiscClampingParallel  PCopyVariant=Disabled  TRVariant=Disabled  FdbkBlocksVariant=Forward  IdealPFdbkVariant=Disabled  SatFdbkVariant=Disabled  DerivativeFilterVariant=Disabled  NVariant=Disabled  NCopyVariant=Disabled_SignalSpec  FilterICVariant=Disabled  IntegratorICVariant=InternalICs  ExternalResetVariant=Disabled  TRSumVariant=Passthrough  SumFdbkVariant=Disabled  SumVariant=Sum_PI  TsampFilterVariant=InternalTs  TsampNgainVariant=Passthrough  TsampIntegralVariant=Disabled_SignalSpec  ExternalSaturationOutDataTypeStr=Inherit: Same as second input
  PID Controller1 : slpidlib/PID Controller  Controller=PI  Form=Parallel  TimeDomain=Discrete-time  UseExternalTs=off  SampleTime=Ts_Control  IntegratorMethod=Forward Euler  FilterMethod=Forward Euler  ControllerParametersSource=internal  P=Kp_Idq  I=Ki_Idq  UseKiTs=off  D=0  N=100  UseFilter=on  TunerSelectOption=Transfer Function Based (PID Tuner App)  InitialConditionSource=internal  InitialConditionForIntegrator=0  InitialConditionForFilter=0  DifferentiatorICPrevScaledInput=0  ExternalReset=none  TrackingMode=off  Kt=1  LimitOutput=on  SatLimitsSource=internal  UpperSaturationLimit=4  LowerSaturationLimit=-4  LinearizeAsGain=on  AntiWindupMode=clamping  Kb=1  LimitIntegrator=off  UpperIntegratorSaturationLimit=inf  LowerIntegratorSaturationLimit=-inf  POutMin=[]  POutMax=[]  IOutMin=[]  IOutMax=[]  DOutMin=[]  DOutMax=[]  NOutMin=[]  NOutMax=[]  SumOutMin=[]  SumOutMax=[]  SaturationOutMin=[]  SaturationOutMax=[]  PParamMin=[]  PParamMax=[]  IParamMin=[]  IParamMax=[]  DParamMin=[]  DParamMax=[]  NParamMin=[]  NParamMax=[]  KbParamMin=[]  KbParamMax=[]  KtParamMin=[]  KtParamMax=[]  KbOutMin=[]  KbOutMax=[]  KtOutMin=[]  KtOutMax=[]  IntegratorOutMin=[]  IntegratorOutMax=[]  FilterOutMin=[]  FilterOutMax=[]  SumI1OutMin=[]  SumI1OutMax=[]  SumI2OutMin=[]  SumI2OutMax=[]  SumI3OutMin=[]  SumI3OutMax=[]  SumI4OutMin=[]  SumI4OutMax=[]  SumDOutMin=[]  SumDOutMax=[]  DifferentiatorOutMin=[]  DifferentiatorOutMax=[]  FilterDiffOutCoefMin=[]  FilterDiffOutCoefMax=[]  ReciprocalOutMin=[]  ReciprocalOutMax=[]  SumDenOutMin=[]  SumDenOutMax=[]  SumNumOutMin=[]  SumNumOutMax=[]  DivideOutMin=[]  DivideOutMax=[]  UdiffTsProdOutMin=[]  UdiffTsProdOutMax=[]  NTsProdOutMin=[]  NTsProdOutMax=[]  UintegralTsProdOutMin=[]  UintegralTsProdOutMax=[]  UngainTsProdOutMin=[]  UngainTsProdOutMax=[]  ClampingZeroOutDataTypeStr=Inherit: Inherit via back propagation  ClampingZeroOutMin=[]  ClampingZeroOutMax=[]  FilterDenConstantOutDataTypeStr=Inherit: Inherit via back propagation  FilterDenConstantOutMin=[]  FilterDenConstantOutMax=[]  PCopyOutDataTypeStr=Inherit: Inherit via back propagation  PCopyOutMin=[]  PCopyOutMax=[]  NCopyOutDataTypeStr=Inherit: Inherit via back propagation  NCopyOutMin=[]  NCopyOutMax=[]  IntegratorContinuousStateAttributes=''  IntegratorStateMustResolveToSignalObject=off  IntegratorRTWStateStorageClass=Auto  FilterContinuousStateAttributes=''  FilterStateMustResolveToSignalObject=off  FilterRTWStateStorageClass=Auto  ParallelPVariant=InternalParameters  IdealPVariant=Disabled  IVariant=InternalParameters  DVariant=Disabled  IntegratorVariant=Discrete  SatVariant=Enabled  AWVariant=DiscClampingParallel  PCopyVariant=Disabled  TRVariant=Disabled  FdbkBlocksVariant=Forward  IdealPFdbkVariant=Disabled  SatFdbkVariant=Disabled  DerivativeFilterVariant=Disabled  NVariant=Disabled  NCopyVariant=Disabled_SignalSpec  FilterICVariant=Disabled  IntegratorICVariant=InternalICs  ExternalResetVariant=Disabled  TRSumVariant=Passthrough  SumFdbkVariant=Disabled  SumVariant=Sum_PI  TsampFilterVariant=InternalTs  TsampNgainVariant=Passthrough  TsampIntegralVariant=Disabled_SignalSpec  ExternalSaturationOutDataTypeStr=Inherit: Same as second input
  Scope : Scope  NumInputPorts=4
  Scope1 : Scope  NumInputPorts=4
  Sum : Sum  Inputs=-+  InputSameDT=on  SaturateOnIntegerOverflow=on  OutDataTypeStr=Inherit: Same as first input
  Sum1 : Sum  Inputs=+-  InputSameDT=on  SaturateOnIntegerOverflow=on  OutDataTypeStr=Inherit: Same as first input
  Sum2 : Sum  Inputs=+--  InputSameDT=on  SaturateOnIntegerOverflow=on  OutDataTypeStr=Inherit: Same as first input
  Sum3 : Sum  Inputs=+-+  InputSameDT=on  SaturateOnIntegerOverflow=on  OutDataTypeStr=Inherit: Same as first input
  UdUq_n : Outport
  wires:
  Sum3/1 -> Mux/2, Scope1/4
  Gain6/1 -> PID Controller/1
  Sum1/1 -> Gain7/1
  Sum2/1 -> Scope/4, Mux/1
  Uc/1 -> Gain2/1
  IdIq_n_Ref/1 -> Demux1/1
  Gain2/1 -> Divide/2
  Gain/1 -> Gain3/1
  Gain1/1 -> Gain5/1
  Edq_n/1 -> Demux2/1
  Gain3/1 -> Sum2/3, Scope/3
  Gain5/1 -> Sum3/3, Scope1/3
  Mux/1 -> Gain4/1
  Divide/1 -> UdUq_n/1
  PID Controller/1 -> Sum2/2, Scope/2
  PID Controller1/1 -> Sum3/2, Scope1/2
  Gain4/1 -> Divide/1
  Sum/1 -> Gain6/1
  Gain7/1 -> PID Controller1/1
  Demux2/1 -> [Ed]
  Demux2/2 -> [Eq]
  [Ed] -> Sum2/1, Scope/1
  [Eq] -> Scope1/1, Sum3/1
  Demux1/1 -> Sum/2
  Demux1/2 -> Sum1/1
  Demux3/2 -> [Iq]
  Demux3/1 -> [Id]
  Idq_n/1 -> Demux3/1
  [Id] -> Sum/1
  [Iq] -> Sum1/2
  [Iq] -> Gain/1
  [Id] -> Gain1/1

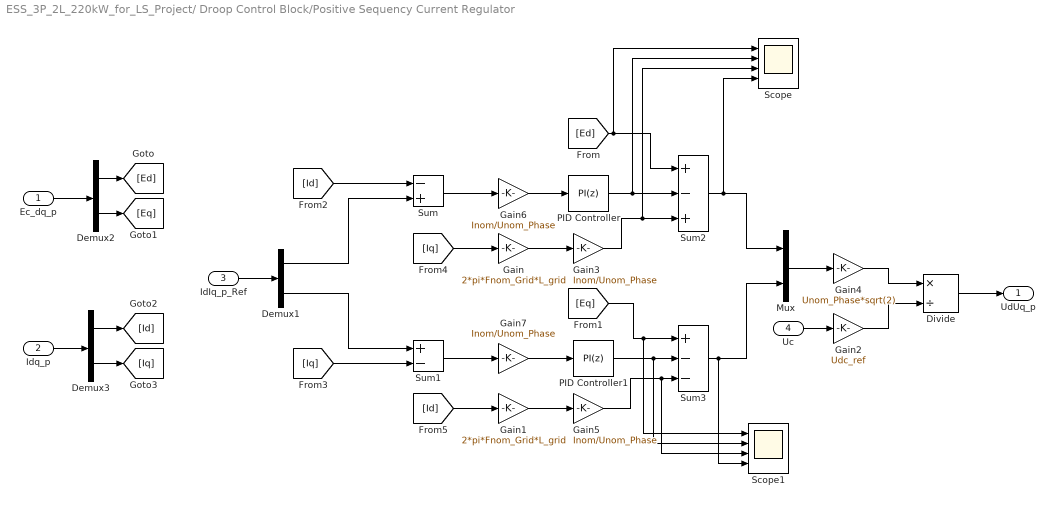
== system ESS_3P_2L_220kW_for_LS_Project/ Droop Control Block/Positive Sequency Current Regulator ==
  Ec_dq_p : Inport
  Idq_p : Inport  Port=2
  IdIq_p_Ref : Inport  Port=3  PortDimensions=2
  Uc : Inport  Port=4
  Demux1 : Demux  Outputs=2
  Demux2 : Demux  Outputs=2
  Demux3 : Demux  Outputs=2
  Divide : Product  Inputs=*/
  Gain : Gain  Gain=2*pi*Fnom_Grid*L_grid
  Gain1 : Gain  Gain=2*pi*Fnom_Grid*L_grid
  Gain2 : Gain  Gain=Udc_ref
  Gain{3,5..7} (4 alike) : Gain  Gain=Inom/Unom_Phase
  Gain4 : Gain  Gain=Unom_Phase*sqrt(2)
  Mux : Mux  Inputs=2
  PID Controller : slpidlib/PID Controller  Controller=PI  Form=Parallel  TimeDomain=Discrete-time  UseExternalTs=off  SampleTime=Ts_Control  IntegratorMethod=Forward Euler  FilterMethod=Forward Euler  ControllerParametersSource=internal  P=Kp_Idq  I=Ki_Idq  UseKiTs=off  D=0  N=100  UseFilter=on  TunerSelectOption=Transfer Function Based (PID Tuner App)  InitialConditionSource=internal  InitialConditionForIntegrator=0  InitialConditionForFilter=0  DifferentiatorICPrevScaledInput=0  ExternalReset=none  TrackingMode=off  Kt=1  LimitOutput=on  SatLimitsSource=internal  UpperSaturationLimit=4  LowerSaturationLimit=-4  LinearizeAsGain=on  AntiWindupMode=clamping  Kb=1  LimitIntegrator=off  UpperIntegratorSaturationLimit=inf  LowerIntegratorSaturationLimit=-inf  POutMin=[]  POutMax=[]  IOutMin=[]  IOutMax=[]  DOutMin=[]  DOutMax=[]  NOutMin=[]  NOutMax=[]  SumOutMin=[]  SumOutMax=[]  SaturationOutMin=[]  SaturationOutMax=[]  PParamMin=[]  PParamMax=[]  IParamMin=[]  IParamMax=[]  DParamMin=[]  DParamMax=[]  NParamMin=[]  NParamMax=[]  KbParamMin=[]  KbParamMax=[]  KtParamMin=[]  KtParamMax=[]  KbOutMin=[]  KbOutMax=[]  KtOutMin=[]  KtOutMax=[]  IntegratorOutMin=[]  IntegratorOutMax=[]  FilterOutMin=[]  FilterOutMax=[]  SumI1OutMin=[]  SumI1OutMax=[]  SumI2OutMin=[]  SumI2OutMax=[]  SumI3OutMin=[]  SumI3OutMax=[]  SumI4OutMin=[]  SumI4OutMax=[]  SumDOutMin=[]  SumDOutMax=[]  DifferentiatorOutMin=[]  DifferentiatorOutMax=[]  FilterDiffOutCoefMin=[]  FilterDiffOutCoefMax=[]  ReciprocalOutMin=[]  ReciprocalOutMax=[]  SumDenOutMin=[]  SumDenOutMax=[]  SumNumOutMin=[]  SumNumOutMax=[]  DivideOutMin=[]  DivideOutMax=[]  UdiffTsProdOutMin=[]  UdiffTsProdOutMax=[]  NTsProdOutMin=[]  NTsProdOutMax=[]  UintegralTsProdOutMin=[]  UintegralTsProdOutMax=[]  UngainTsProdOutMin=[]  UngainTsProdOutMax=[]  ClampingZeroOutDataTypeStr=Inherit: Inherit via back propagation  ClampingZeroOutMin=[]  ClampingZeroOutMax=[]  FilterDenConstantOutDataTypeStr=Inherit: Inherit via back propagation  FilterDenConstantOutMin=[]  FilterDenConstantOutMax=[]  PCopyOutDataTypeStr=Inherit: Inherit via back propagation  PCopyOutMin=[]  PCopyOutMax=[]  NCopyOutDataTypeStr=Inherit: Inherit via back propagation  NCopyOutMin=[]  NCopyOutMax=[]  IntegratorContinuousStateAttributes=''  IntegratorStateMustResolveToSignalObject=off  IntegratorRTWStateStorageClass=Auto  FilterContinuousStateAttributes=''  FilterStateMustResolveToSignalObject=off  FilterRTWStateStorageClass=Auto  ParallelPVariant=InternalParameters  IdealPVariant=Disabled  IVariant=InternalParameters  DVariant=Disabled  IntegratorVariant=Discrete  SatVariant=Enabled  AWVariant=DiscClampingParallel  PCopyVariant=Disabled  TRVariant=Disabled  FdbkBlocksVariant=Forward  IdealPFdbkVariant=Disabled  SatFdbkVariant=Disabled  DerivativeFilterVariant=Disabled  NVariant=Disabled  NCopyVariant=Disabled_SignalSpec  FilterICVariant=Disabled  IntegratorICVariant=InternalICs  ExternalResetVariant=Disabled  TRSumVariant=Passthrough  SumFdbkVariant=Disabled  SumVariant=Sum_PI  TsampFilterVariant=InternalTs  TsampNgainVariant=Passthrough  TsampIntegralVariant=Disabled_SignalSpec  ExternalSaturationOutDataTypeStr=Inherit: Same as second input
  PID Controller1 : slpidlib/PID Controller  Controller=PI  Form=Parallel  TimeDomain=Discrete-time  UseExternalTs=off  SampleTime=Ts_Control  IntegratorMethod=Forward Euler  FilterMethod=Forward Euler  ControllerParametersSource=internal  P=Kp_Idq  I=Ki_Idq  UseKiTs=off  D=0  N=100  UseFilter=on  TunerSelectOption=Transfer Function Based (PID Tuner App)  InitialConditionSource=internal  InitialConditionForIntegrator=0  InitialConditionForFilter=0  DifferentiatorICPrevScaledInput=0  ExternalReset=none  TrackingMode=off  Kt=1  LimitOutput=on  SatLimitsSource=internal  UpperSaturationLimit=4  LowerSaturationLimit=-4  LinearizeAsGain=on  AntiWindupMode=clamping  Kb=1  LimitIntegrator=off  UpperIntegratorSaturationLimit=inf  LowerIntegratorSaturationLimit=-inf  POutMin=[]  POutMax=[]  IOutMin=[]  IOutMax=[]  DOutMin=[]  DOutMax=[]  NOutMin=[]  NOutMax=[]  SumOutMin=[]  SumOutMax=[]  SaturationOutMin=[]  SaturationOutMax=[]  PParamMin=[]  PParamMax=[]  IParamMin=[]  IParamMax=[]  DParamMin=[]  DParamMax=[]  NParamMin=[]  NParamMax=[]  KbParamMin=[]  KbParamMax=[]  KtParamMin=[]  KtParamMax=[]  KbOutMin=[]  KbOutMax=[]  KtOutMin=[]  KtOutMax=[]  IntegratorOutMin=[]  IntegratorOutMax=[]  FilterOutMin=[]  FilterOutMax=[]  SumI1OutMin=[]  SumI1OutMax=[]  SumI2OutMin=[]  SumI2OutMax=[]  SumI3OutMin=[]  SumI3OutMax=[]  SumI4OutMin=[]  SumI4OutMax=[]  SumDOutMin=[]  SumDOutMax=[]  DifferentiatorOutMin=[]  DifferentiatorOutMax=[]  FilterDiffOutCoefMin=[]  FilterDiffOutCoefMax=[]  ReciprocalOutMin=[]  ReciprocalOutMax=[]  SumDenOutMin=[]  SumDenOutMax=[]  SumNumOutMin=[]  SumNumOutMax=[]  DivideOutMin=[]  DivideOutMax=[]  UdiffTsProdOutMin=[]  UdiffTsProdOutMax=[]  NTsProdOutMin=[]  NTsProdOutMax=[]  UintegralTsProdOutMin=[]  UintegralTsProdOutMax=[]  UngainTsProdOutMin=[]  UngainTsProdOutMax=[]  ClampingZeroOutDataTypeStr=Inherit: Inherit via back propagation  ClampingZeroOutMin=[]  ClampingZeroOutMax=[]  FilterDenConstantOutDataTypeStr=Inherit: Inherit via back propagation  FilterDenConstantOutMin=[]  FilterDenConstantOutMax=[]  PCopyOutDataTypeStr=Inherit: Inherit via back propagation  PCopyOutMin=[]  PCopyOutMax=[]  NCopyOutDataTypeStr=Inherit: Inherit via back propagation  NCopyOutMin=[]  NCopyOutMax=[]  IntegratorContinuousStateAttributes=''  IntegratorStateMustResolveToSignalObject=off  IntegratorRTWStateStorageClass=Auto  FilterContinuousStateAttributes=''  FilterStateMustResolveToSignalObject=off  FilterRTWStateStorageClass=Auto  ParallelPVariant=InternalParameters  IdealPVariant=Disabled  IVariant=InternalParameters  DVariant=Disabled  IntegratorVariant=Discrete  SatVariant=Enabled  AWVariant=DiscClampingParallel  PCopyVariant=Disabled  TRVariant=Disabled  FdbkBlocksVariant=Forward  IdealPFdbkVariant=Disabled  SatFdbkVariant=Disabled  DerivativeFilterVariant=Disabled  NVariant=Disabled  NCopyVariant=Disabled_SignalSpec  FilterICVariant=Disabled  IntegratorICVariant=InternalICs  ExternalResetVariant=Disabled  TRSumVariant=Passthrough  SumFdbkVariant=Disabled  SumVariant=Sum_PI  TsampFilterVariant=InternalTs  TsampNgainVariant=Passthrough  TsampIntegralVariant=Disabled_SignalSpec  ExternalSaturationOutDataTypeStr=Inherit: Same as second input
  Scope : Scope  NumInputPorts=4
  Scope1 : Scope  NumInputPorts=4
  Sum : Sum  Inputs=-+  InputSameDT=on  SaturateOnIntegerOverflow=on  OutDataTypeStr=Inherit: Same as first input
  Sum1 : Sum  Inputs=+-  InputSameDT=on  SaturateOnIntegerOverflow=on  OutDataTypeStr=Inherit: Same as first input
  Sum2 : Sum  Inputs=+-+  InputSameDT=on  SaturateOnIntegerOverflow=on  OutDataTypeStr=Inherit: Same as first input
  Sum3 : Sum  Inputs=+--  InputSameDT=on  SaturateOnIntegerOverflow=on  OutDataTypeStr=Inherit: Same as first input
  UdUq_p : Outport
  wires:
  Gain6/1 -> PID Controller/1
  PID Controller/1 -> Sum2/2, Scope/2
  [Id] -> Gain1/1
  [Iq] -> Gain/1
  [Iq] -> Sum1/2
  [Id] -> Sum/1
  Idq_p/1 -> Demux3/1
  Demux3/1 -> [Id]
  Demux3/2 -> [Iq]
  Demux1/2 -> Sum1/1
  Demux1/1 -> Sum/2
  [Eq] -> Scope1/1, Sum3/1
  [Ed] -> Sum2/1, Scope/1
  Demux2/2 -> [Eq]
  Demux2/1 -> [Ed]
  Gain7/1 -> PID Controller1/1
  Sum/1 -> Gain6/1
  Gain4/1 -> Divide/1
  PID Controller1/1 -> Sum3/2, Scope1/2
  Divide/1 -> UdUq_p/1
  Mux/1 -> Gain4/1
  Gain5/1 -> Sum3/3, Scope1/3
  Gain3/1 -> Sum2/3, Scope/3
  Ec_dq_p/1 -> Demux2/1
  Gain1/1 -> Gain5/1
  Gain/1 -> Gain3/1
  Gain2/1 -> Divide/2
  IdIq_p_Ref/1 -> Demux1/1
  Uc/1 -> Gain2/1
  Sum2/1 -> Mux/1, Scope/4
  Sum1/1 -> Gain7/1
  Sum3/1 -> Mux/2, Scope1/4
